simulink model "Foc"  (R2025b)
settings: Solver=FixedStepDiscrete  StartTime=0.0  StopTime=10.0  FixedStep=0.001  RelTol=1e-3
values from neighbouring files (symbols this model uses):
  cal_bActHwMode = NoneSAR.Parameter    [Foc_2024b_LoadCalParameter.m]    (also in Foc_LoadCalParameter.m)
  cal_f32AdcMaxCountsHw = NoneSAR.Parameter    [Foc_LoadCalParameter.m]
  cal_f32AdcRefVoltHw = NoneSAR.Parameter    [Foc_LoadCalParameter.m]
  cal_f32AdcVoltMidHw = NoneSAR.Parameter    [Foc_LoadCalParameter.m]
  cal_f32FullScaleCur = NoneSAR.Parameter    [Foc_LoadCalParameter.m]
  cal_f32GainAmpHw = NoneSAR.Parameter    [Foc_LoadCalParameter.m]
  cal_f32OhmRShuntHw = NoneSAR.Parameter    [Foc_LoadCalParameter.m]
  cal_s16HwtDutyU = NoneSAR.Parameter    [Foc_LoadCalParameter.m]
  cal_s16HwtDutyV = NoneSAR.Parameter    [Foc_LoadCalParameter.m]
  cal_s16HwtDutyW = NoneSAR.Parameter    [Foc_LoadCalParameter.m]
  cal_s16IdKi = NoneSAR.Parameter    [Foc_LoadCalParameter.m]
  cal_s16IdKp = NoneSAR.Parameter    [Foc_LoadCalParameter.m]
  cal_s16IdMaxOut = NoneSAR.Parameter    [Foc_LoadCalParameter.m]
  cal_s16IdMinOut = NoneSAR.Parameter    [Foc_LoadCalParameter.m]
  cal_s16Inductivity = NoneSAR.Parameter    [Foc_2024b_LoadCalParameter.m]    (also in Foc_LoadCalParameter.m)
  cal_s16IqKi = NoneSAR.Parameter    [Foc_LoadCalParameter.m]
  cal_s16IqKp = NoneSAR.Parameter    [Foc_LoadCalParameter.m]
  cal_s16IqMaxOut = NoneSAR.Parameter    [Foc_LoadCalParameter.m]
  cal_s16IqMinOut = NoneSAR.Parameter    [Foc_LoadCalParameter.m]
  cal_s16LpfPllEst = NoneSAR.Parameter    [Foc_2024b_LoadCalParameter.m]    (also in Foc_LoadCalParameter.m)
  cal_s16LpfPllEstOpenLoop = NoneSAR.Parameter    [Foc_2024b_LoadCalParameter.m]    (also in Foc_LoadCalParameter.m)
  cal_s16MinSampleTime = NoneSAR.Parameter    [Foc_2024b_LoadCalParameter.m]    (also in Foc_LoadCalParameter.m)
  cal_s16OmegaGainEst = NoneSAR.Parameter    [Foc_2024b_LoadCalParameter.m]    (also in Foc_LoadCalParameter.m)
  cal_s16RPha = NoneSAR.Parameter    [Foc_2024b_LoadCalParameter.m]    (also in Foc_LoadCalParameter.m)
  cal_s16ThresholdPhaCurImplaisible = NoneSAR.Parameter    [Foc_2024b_LoadCalParameter.m]    (also in Foc_LoadCalParameter.m)
  cal_s8IdFacKi = NoneSAR.Parameter    [Foc_LoadCalParameter.m]
  cal_s8IdFacKp = NoneSAR.Parameter    [Foc_LoadCalParameter.m]
  cal_s8IqFacKi = NoneSAR.Parameter    [Foc_LoadCalParameter.m]
  cal_s8IqFacKp = NoneSAR.Parameter    [Foc_LoadCalParameter.m]
  cal_u16AdcTriggerOffset = NoneSAR.Parameter    [Foc_LoadCalParameter.m]
  cal_u8HwtSector = NoneSAR.Parameter    [Foc_LoadCalParameter.m]
  cal_u8TiDebPhaCur = NoneSAR.Parameter    [Foc_2024b_LoadCalParameter.m]    (also in Foc_LoadCalParameter.m)
undefined symbols (not defined in the file or in its folder): CCU6_T12PERIOD, CCU_PWM_PERIOD_TICKS_HALF, DCLINK_VOLTAGE_FACTOR, DesiredPwm_U, DesiredPwm_V, DesiredPwm_W, e_motorstate_t, e_running_dir_t, FOC_SVM_MAX, FOC_VD_VQ_MAX, FOC_VD_VQ_MAX_100, FOC_VD_VQ_MAX_95, FOC_VD_VQ_MAX_97, FOCLLD_CCU_PWM_PERIOD_TICKS_HALF, FOCLLD_SKIP_DEAD_TIME_THRESHOLD, MAX_DUTY, MIN_SAMPLE_TIME_DEFAULT, MODULATION_FLATBOTTOM, ONEBY_CURRENT_AMPLIFICATION, PhaseCurrentU, PhaseCurrentV, PhaseCurrentW, PwmShift_DutyLong, PwmShift_DutyMed, PwmShift_DutyShort, PwmShiftPtr_RiseLong, PwmShiftPtr_RiseMed, PwmShiftPtr_RiseShort, s16_EST_THETA_GAIN, s16_ONEBYSQR3, s16_SQR3OVER2, st_c_pi_Q_s16_outMax, st_c_pi_Q_s16_outMin, U8_INDUCTIVITY_FAC, VQ_MAX_TABLE_SIZE, VqMaxTable_100, VqMaxTable_95, VqMaxTable_97
libraries: simulink x16, hdlsllib x2
(part 2 of 6)

== system Foc/FieldOrientedControl/CurrentControl/MOTOR_STATE_CLOSED_LOOP ==
  s16ThetaEst : Inport  OutDataTypeStr=int16
  s16Id : Inport  Port=2  OutDataTypeStr=int16
  s16Iq : Inport  Port=3  OutDataTypeStr=int16
  bEnMotorDriverLast : Inport  Port=4  OutDataTypeStr=boolean
  s16IdRef : Inport  Port=5  OutDataTypeStr=int16
  s16IqRef : Inport  Port=6  OutDataTypeStr=int16
  IqPiBus : Inport  Port=7
  IdPiBus : Inport  Port=8
  " PiCtrl_Calc" : Subsystem
  Bus Creator : BusCreator  Inputs=4
  PIControl_update : Subsystem
  foc_state : Outport
  wires:
  Bus Creator/1 -> foc_state/1
  s16Id/1 -> " PiCtrl_Calc"/1(s16Id)
  s16Iq/1 -> PIControl_update/1(s16Iq)
  PIControl_update/1(s16Vq) -> Bus Creator/3  "s16Vq"
  s16ThetaEst/1 -> Bus Creator/1  "s16_foc_parkangle"
  " PiCtrl_Calc"/1(s16Vd) -> Bus Creator/2  "s16Vd"
  bEnMotorDriverLast/1 -> Bus Creator/4  "bEnMotorDriver"
  s16IdRef/1 -> " PiCtrl_Calc"/2(s16IdRef)
  IdPiBus/1 -> " PiCtrl_Calc"/3(IdPiBus)
  s16IqRef/1 -> PIControl_update/2(s16IqRef)
  IqPiBus/1 -> PIControl_update/3(IqPiBus)

== system Foc/FieldOrientedControl/CurrentControl/MOTOR_STATE_RAMP ==
  eDirRun : Inport
  s16AngleParkLast : Inport  Port=2  OutDataTypeStr=int16
  s16Id : Inport  Port=3  OutDataTypeStr=int16
  s16Iq : Inport  Port=4  OutDataTypeStr=int16
  bEnMotorDriverLast : Inport  Port=5  OutDataTypeStr=boolean
  u32SpdRamp : Inport  Port=6  OutDataTypeStr=uint32
  s16IdRef : Inport  Port=7  OutDataTypeStr=int16
  s16IqRef : Inport  Port=8  OutDataTypeStr=int16
  IqPiBus : Inport  Port=9
  IdPiBus : Inport  Port=10
  Bus Creator : BusCreator  Inputs=4
  PiCtrl_Calc_D : Subsystem
  "PiCtrl_Calc_Q " : Subsystem
  parkangle_cal : Subsystem
  foc_state : Outport
  wires:
  eDirRun/1 -> parkangle_cal/1(eDirRun)
  u32SpdRamp/1 -> parkangle_cal/2(u32SpdRamp)
  PiCtrl_Calc_D/1(s16Vd) -> Bus Creator/2  "s16_foc_v_d"
  s16AngleParkLast/1 -> parkangle_cal/3(s16AngleParkLast)
  s16Id/1 -> PiCtrl_Calc_D/1(s16Id)
  parkangle_cal/1(s16AnglePark) -> Bus Creator/1  "s16_foc_parkangle"
  s16Iq/1 -> "PiCtrl_Calc_Q "/1(s16Iq)
  "PiCtrl_Calc_Q "/1(s16Vq) -> Bus Creator/3  "s16_foc_v_q"
  bEnMotorDriverLast/1 -> Bus Creator/4  "bEnMotorDriver"
  Bus Creator/1 -> foc_state/1
  s16IdRef/1 -> PiCtrl_Calc_D/2(s16IdRef)
  IdPiBus/1 -> PiCtrl_Calc_D/3(IdPiBus)
  s16IqRef/1 -> "PiCtrl_Calc_Q "/2(s16IqRef)
  IqPiBus/1 -> "PiCtrl_Calc_Q "/3(IqPiBus)

== system Foc/FieldOrientedControl/CurrentControl/MOTOR_STATE_RAMP_INIT ==
  s16AngleParkLast : Inport  OutDataTypeStr=int16
  s16Id : Inport  Port=2  OutDataTypeStr=int16
  s16Iq : Inport  Port=3  OutDataTypeStr=int16
  bEnMotorDriverLast : Inport  Port=4  OutDataTypeStr=boolean
  s16IdRef : Inport  Port=5  OutDataTypeStr=int16
  s16IqRef : Inport  Port=6  OutDataTypeStr=int16
  IqPiBus : Inport  Port=7
  IdPiBus : Inport  Port=8
  Compare To Constant : simulink/Logic and Bit Operations/Compare To Constant  relop===  const=false  OutDataTypeStr=boolean
  EnableDriver : Subsystem
  SetPiController : Subsystem
  Switch : Switch  Criteria=u2 ~= 0  SaturateOnIntegerOverflow=off  InputSameDT=off
  foc_state : Outport
  wires:
  s16AngleParkLast/1 -> EnableDriver/1(s16AngleParkLast)
  s16Id/1 -> SetPiController/1(s16Id)
  bEnMotorDriverLast/1 -> SetPiController/3(bEnMotorDriverLast), Compare To Constant/1
  s16Iq/1 -> SetPiController/2(s16Iq)
  EnableDriver/1(foc_state) -> Switch/1
  Compare To Constant/1 -> Switch/2
  SetPiController/1(foc_state) -> Switch/3
  Switch/1 -> foc_state/1
  s16IdRef/1 -> SetPiController/4(s16IdRef)
  IdPiBus/1 -> SetPiController/7(IdPiBus)
  s16IqRef/1 -> SetPiController/5(s16IqRef)
  IqPiBus/1 -> SetPiController/6(IqPiBus)

== system Foc/FieldOrientedControl/CurrentControl/default ==
  bEnMotorDriverLast : Inport  OutDataTypeStr=boolean
  Bus Creator : BusCreator  Inputs=4
  Constant : Constant  Value=0  OutDataTypeStr=fixdt(1,16,15)
  Constant1 : Constant  Value=0  OutDataTypeStr=fixdt(1,16,15)
  Constant2 : Constant  Value=0  OutDataTypeStr=fixdt(1,16,15)
  foc_state : Outport
  wires:
  Constant/1 -> Bus Creator/1  "s16AnglePark"
  Constant1/1 -> Bus Creator/2  "s16Vd"
  Constant2/1 -> Bus Creator/3  "s16Vq"
  bEnMotorDriverLast/1 -> Bus Creator/4  "bEnMotorDriver"
  Bus Creator/1 -> foc_state/1

== system Foc/FieldOrientedControl/CurrentOffsets/OffsetDefault ==
  Action Port : ActionPort  ActionPortLabel=else
  Constant1 : Constant  Value=0  OutDataTypeStr=int32
  Constant2 : Constant  Value=0  OutDataTypeStr=int16
  Constant3 : Constant  Value=0  OutDataTypeStr=int16
  Constant4 : Constant  Value=0  OutDataTypeStr=int32
  s16PhaCurU : Outport  OutDataTypeStr=int16
  s16PhaCurV : Outport  Port=2  OutDataTypeStr=int16
  s32CurOffsetU : Outport  Port=3  OutDataTypeStr=int32
  s32CurOffsetV : Outport  Port=4  OutDataTypeStr=int32
  wires:
  Constant3/1 -> s16PhaCurV/1
  Constant4/1 -> s32CurOffsetV/1
  Constant1/1 -> s32CurOffsetU/1
  Constant2/1 -> s16PhaCurU/1

== system Foc/FieldOrientedControl/CurrentOffsets/OffsetDetection ==
  s16PhaCurRawU : Inport  OutDataTypeStr=int16
  s16PhaCurRawV : Inport  Port=2  OutDataTypeStr=int16
  s32CurOffsetULast : Inport  Port=3  OutDataTypeStr=int32
  s32CurOffsetVLast : Inport  Port=4  OutDataTypeStr=int32
  Action Port : ActionPort  ActionPortLabel=if(u1)
  Add : Sum  Inputs=+-  OutDataTypeStr=fixdt(1,16,15)
  Add1 : Sum  Inputs=+-  OutDataTypeStr=fixdt(1,16,15)
  Add2 : Sum  OutDataTypeStr=int32
  Add3 : Sum  OutDataTypeStr=int32
  Bit Shift : hdlsllib/Logic and Bit Operations/Bit Shift  mode=Shift Right Logical  N=16
  Bit Shift1 : hdlsllib/Logic and Bit Operations/Bit Shift  mode=Shift Right Logical  N=16
  Data Type Conversion : DataTypeConversion  OutDataTypeStr=int16  SaturateOnIntegerOverflow=off  RndMeth=Floor
  Data Type Conversion1 : DataTypeConversion  OutDataTypeStr=int16  SaturateOnIntegerOverflow=off  RndMeth=Floor
  s16PhaCurU : Outport  OutDataTypeStr=int16
  s16PhaCurV : Outport  Port=2  OutDataTypeStr=int16
  s32CurOffsetU : Outport  Port=3  OutDataTypeStr=int32
  s32CurOffsetV : Outport  Port=4  OutDataTypeStr=int32
  wires:
  s32CurOffsetVLast/1 -> Add3/2, Bit Shift1/1
  s16PhaCurRawV/1 -> Add1/1
  s32CurOffsetULast/1 -> Add2/2, Bit Shift/1
  s16PhaCurRawU/1 -> Add/1
  Bit Shift/1 -> Data Type Conversion1/1
  Data Type Conversion/1 -> Add1/2
  Data Type Conversion1/1 -> Add/2
  Bit Shift1/1 -> Data Type Conversion/1
  Add3/1 -> s32CurOffsetV/1
  Add2/1 -> s32CurOffsetU/1
  Add1/1 -> Add3/1, s16PhaCurV/1
  Add/1 -> s16PhaCurU/1, Add2/1

== system Foc/FieldOrientedControl/GetCurrents/AdcVolToCur ==
  u16SsCur1 : Inport  OutDataTypeStr=uint16
  u16SsCur2 : Inport  Port=2  OutDataTypeStr=uint16
  Add : Sum  Inputs=+-
  Add1 : Sum
  Add2 : Sum  Inputs=+-
  Add3 : Sum
  Constant : Constant  Value=cal_f32AdcMaxCountsHw  OutDataTypeStr=single
  Constant1 : Constant  Value=cal_f32AdcRefVoltHw  OutDataTypeStr=single
  Constant10 : Constant  Value=cal_f32AdcRefVoltHw  OutDataTypeStr=single
  Constant11 : Constant  Value=cal_f32OhmRShuntHw  OutDataTypeStr=single
  Constant12 : Constant  Value=cal_f32GainAmpHw  OutDataTypeStr=single
  Constant13 : Constant  Value=cal_f32AdcVoltMidHw  OutDataTypeStr=single
  Constant14 : Constant  Value=0.5  OutDataTypeStr=single
  Constant15 : Constant  Value=-0.5  OutDataTypeStr=single
  Constant16 : Constant  Value=32767  OutDataTypeStr=single
  Constant17 : Constant  Value=cal_f32FullScaleCur  OutDataTypeStr=single
  Constant2 : Constant  Value=cal_f32OhmRShuntHw  OutDataTypeStr=single
  Constant3 : Constant  Value=cal_f32GainAmpHw  OutDataTypeStr=single
  Constant4 : Constant  Value=cal_f32AdcVoltMidHw  OutDataTypeStr=single
  Constant5 : Constant  Value=0.5  OutDataTypeStr=single
  Constant6 : Constant  Value=-0.5  OutDataTypeStr=single
  Constant7 : Constant  Value=32767  OutDataTypeStr=single
  Constant8 : Constant  Value=cal_f32FullScaleCur  OutDataTypeStr=single
  Constant9 : Constant  Value=cal_f32AdcMaxCountsHw  OutDataTypeStr=single
  Data Type Conversion : DataTypeConversion  OutDataTypeStr=single  SaturateOnIntegerOverflow=off  RndMeth=Floor
  Data Type Conversion1 : DataTypeConversion  OutDataTypeStr=single  SaturateOnIntegerOverflow=off  RndMeth=Floor
  Data Type Conversion : DataTypeConversion  OutDataTypeStr=int32  SaturateOnIntegerOverflow=off  RndMeth=Floor
  Data Type Conversion1 : DataTypeConversion  OutDataTypeStr=int32  SaturateOnIntegerOverflow=off  RndMeth=Floor
  Divide{,3..4,6,9..10} (6 alike) : Product  Inputs=*/
  Divide{1..2,5,7..8,11} (6 alike) : Product  Inputs=**
  Saturation : Saturate  UpperLimit=32767  LowerLimit=-32768  OutDataTypeStr=int16
  Saturation1 : Saturate  UpperLimit=32767  LowerLimit=-32768  OutDataTypeStr=int16
  Switch : Switch  Criteria=u2 > Threshold  SaturateOnIntegerOverflow=off  InputSameDT=off
  Switch1 : Switch  Criteria=u2 > Threshold  SaturateOnIntegerOverflow=off  InputSameDT=off
  s16SsCur1 : Outport  OutDataTypeStr=int16
  s16SsCur2 : Outport  Port=2  OutDataTypeStr=int16
  wires:
  u16SsCur1/1 -> Data Type Conversion/1
  Add1/1 -> Data Type Conversion/1
  Add3/1 -> Data Type Conversion1/1
  u16SsCur2/1 -> Data Type Conversion1/1
  Data Type Conversion/1 -> Divide/1
  Divide10/1 -> Divide11/1
  Divide/1 -> Divide1/1
  Constant9/1 -> Divide6/2
  Constant8/1 -> Divide4/2
  Data Type Conversion1/1 -> Divide6/1
  Constant6/1 -> Switch/3
  Constant14/1 -> Switch1/1
  Constant2/1 -> Divide2/1
  Constant10/1 -> Divide7/2
  Constant16/1 -> Divide11/2
  Constant4/1 -> Add/2
  Constant12/1 -> Divide8/2
  Constant/1 -> Divide/2
  Divide4/1 -> Divide5/1
  Divide2/1 -> Divide3/2
  Divide8/1 -> Divide9/2
  Divide6/1 -> Divide7/1
  Constant5/1 -> Switch/1
  Constant17/1 -> Divide10/2
  Constant13/1 -> Add2/2
  Constant1/1 -> Divide1/2
  Divide5/1 -> Add1/2
  Divide3/1 -> Divide4/1, Switch/2
  Divide9/1 -> Switch1/2, Divide10/1
  Divide7/1 -> Add2/1
  Constant7/1 -> Divide5/2
  Constant15/1 -> Switch1/3
  Constant3/1 -> Divide2/2
  Constant11/1 -> Divide8/1
  Data Type Conversion1/1 -> Saturation1/1
  Divide11/1 -> Add3/2
  Divide1/1 -> Add/1
  Add/1 -> Divide3/1
  Add2/1 -> Divide9/1
  Switch1/1 -> Add3/1
  Saturation/1 -> s16SsCur1/1
  Switch/1 -> Add1/1
  Data Type Conversion/1 -> Saturation/1
  Saturation1/1 -> s16SsCur2/1

== system Foc/FieldOrientedControl/GetCurrents/DEFAULT ==
  Action Port : ActionPort
  Constant : Constant  Value=0  OutDataTypeStr=int16
  Constant1 : Constant  Value=0  OutDataTypeStr=int16
  Constant2 : Constant  Value=0  OutDataTypeStr=int16
  s16PhaCurU : Outport  OutDataTypeStr=int16
  s16PhaCurV : Outport  Port=2  OutDataTypeStr=int16
  s16PhaCurW : Outport  Port=3  OutDataTypeStr=int16
  wires:
  Constant1/1 -> s16PhaCurV/1
  Constant/1 -> s16PhaCurW/1
  Constant2/1 -> s16PhaCurU/1

== system Foc/FieldOrientedControl/GetCurrents/SECTOR_1 ==
  s16SsCur1 : Inport  OutDataTypeStr=int16
  s16SsCur2 : Inport  Port=2  OutDataTypeStr=int16
  Action Port : ActionPort
  Add : Sum  Inputs=+-  OutDataTypeStr=fixdt(1,16,15)
  Constant : Constant  Value=-1  OutDataTypeStr=int16
  Gain : Gain  Gain=-1
  Product : Product  OutDataTypeStr=fixdt(1,16,15)
  s16PhaCurU : Outport  OutDataTypeStr=int16
  s16PhaCurV : Outport  Port=2  OutDataTypeStr=int16
  s16PhaCurW : Outport  Port=3  OutDataTypeStr=int16
  wires:
  Add/1 -> s16PhaCurU/1
  Product/1 -> Add/2, s16PhaCurW/1
  Gain/1 -> Add/1
  Constant/1 -> Product/2
  s16SsCur2/1 -> Product/1
  s16SsCur1/1 -> Gain/1, s16PhaCurV/1

== system Foc/FieldOrientedControl/GetCurrents/SECTOR_2 ==
  s16SsCur1 : Inport  OutDataTypeStr=int16
  s16SsCur2 : Inport  Port=2  OutDataTypeStr=int16
  Action Port : ActionPort
  Add : Sum  Inputs=+-  OutDataTypeStr=fixdt(1,16,15)
  Constant : Constant  Value=-1  OutDataTypeStr=int16
  Gain : Gain  Gain=-1
  Product : Product  OutDataTypeStr=fixdt(1,16,15)
  s16PhaCurU : Outport  OutDataTypeStr=int16
  s16PhaCurV : Outport  Port=2  OutDataTypeStr=int16
  s16PhaCurW : Outport  Port=3  OutDataTypeStr=int16
  wires:
  Add/1 -> s16PhaCurW/1
  s16SsCur2/1 -> Product/1
  s16SsCur1/1 -> s16PhaCurU/1, Gain/1
  Product/1 -> s16PhaCurV/1, Add/2
  Gain/1 -> Add/1
  Constant/1 -> Product/2

== system Foc/FieldOrientedControl/GetCurrents/SECTOR_3 ==
  s16SsCur1 : Inport  OutDataTypeStr=int16
  s16SsCur2 : Inport  Port=2  OutDataTypeStr=int16
  Action Port : ActionPort
  Add : Sum  Inputs=+-  OutDataTypeStr=fixdt(1,16,15)
  Constant : Constant  Value=-1  OutDataTypeStr=int16
  Gain : Gain  Gain=-1
  Product : Product  OutDataTypeStr=fixdt(1,16,15)
  s16PhaCurU : Outport  OutDataTypeStr=int16
  s16PhaCurV : Outport  Port=2  OutDataTypeStr=int16
  s16PhaCurW : Outport  Port=3  OutDataTypeStr=int16
  wires:
  Product/1 -> s16PhaCurW/1, Add/2
  Gain/1 -> Add/1
  s16SsCur2/1 -> Product/1
  s16SsCur1/1 -> Gain/1, s16PhaCurU/1
  Add/1 -> s16PhaCurV/1
  Constant/1 -> Product/2

== system Foc/FieldOrientedControl/GetCurrents/SECTOR_4 ==
  s16SsCur1 : Inport  OutDataTypeStr=int16
  s16SsCur2 : Inport  Port=2  OutDataTypeStr=int16
  Action Port : ActionPort
  Add : Sum  Inputs=+-  OutDataTypeStr=fixdt(1,16,15)
  Constant : Constant  Value=-1  OutDataTypeStr=int16
  Gain : Gain  Gain=-1
  Product : Product  OutDataTypeStr=fixdt(1,16,15)
  s16PhaCurU : Outport  OutDataTypeStr=int16
  s16PhaCurV : Outport  Port=2  OutDataTypeStr=int16
  s16PhaCurW : Outport  Port=3  OutDataTypeStr=int16
  wires:
  Product/1 -> s16PhaCurU/1, Add/2
  Gain/1 -> Add/1
  s16SsCur2/1 -> Product/1
  s16SsCur1/1 -> s16PhaCurW/1, Gain/1
  Add/1 -> s16PhaCurV/1
  Constant/1 -> Product/2

== system Foc/FieldOrientedControl/GetCurrents/SECTOR_5 ==
  s16SsCur1 : Inport  OutDataTypeStr=int16
  s16SsCur2 : Inport  Port=2  OutDataTypeStr=int16
  Action Port : ActionPort
  Add : Sum  Inputs=+-  OutDataTypeStr=fixdt(1,16,15)
  Constant : Constant  Value=-1  OutDataTypeStr=int16
  Gain : Gain  Gain=-1
  Product : Product  OutDataTypeStr=fixdt(1,16,15)
  s16PhaCurU : Outport  OutDataTypeStr=int16
  s16PhaCurV : Outport  Port=2  OutDataTypeStr=int16
  s16PhaCurW : Outport  Port=3  OutDataTypeStr=int16
  wires:
  Product/1 -> Add/2, s16PhaCurU/1
  Gain/1 -> Add/1
  s16SsCur2/1 -> Product/1
  s16SsCur1/1 -> s16PhaCurV/1, Gain/1
  Add/1 -> s16PhaCurW/1
  Constant/1 -> Product/2

== system Foc/FieldOrientedControl/GetCurrents/SECTOR_6 ==
  s16SsCur1 : Inport  OutDataTypeStr=int16
  s16SsCur2 : Inport  Port=2  OutDataTypeStr=int16
  Action Port : ActionPort
  Add : Sum  Inputs=+-  OutDataTypeStr=fixdt(1,16,15)
  Constant : Constant  Value=-1  OutDataTypeStr=int16
  Gain : Gain  Gain=-1
  Product : Product  OutDataTypeStr=fixdt(1,16,15)
  s16PhaCurU : Outport  OutDataTypeStr=int16
  s16PhaCurV : Outport  Port=2  OutDataTypeStr=int16
  s16PhaCurW : Outport  Port=3  OutDataTypeStr=int16
  wires:
  s16SsCur2/1 -> Product/1
  s16SsCur1/1 -> s16PhaCurW/1, Gain/1
  Add/1 -> s16PhaCurU/1
  Constant/1 -> Product/2
  Product/1 -> s16PhaCurV/1, Add/2
  Gain/1 -> Add/1

== system Foc/FieldOrientedControl/PhaseCurrentSpikeMonitor/b_fault_debounce  ==
  bSymptom : Inport  OutDataTypeStr=boolean
  u8TiDeb : Inport  Port=2  OutDataTypeStr=uint8
  Add : Sum
  CNST_ONE : Constant  OutDataTypeStr=uint8
  CNST_Thd : Constant  Value=200
  CNST_Thd1 : Constant  Value=200
  CNST_Zero : Constant  Value=0
  CNST_flase : Constant  Value=false  OutDataTypeStr=boolean
  CNST_true : Constant  Value=true  OutDataTypeStr=boolean
  DLY_timer : UnitDelay  SampleTime=-1  HasFrameUpgradeWarning=on
  Relational Operator : RelationalOperator  Operator=<  OutDataTypeStr=boolean  RndMeth=Simplest  InputSameDT=off
  Relational Operator1 : RelationalOperator  OutDataTypeStr=boolean  RndMeth=Simplest  InputSameDT=off
  Switch1 : Switch  Criteria=u2 ~= 0  SaturateOnIntegerOverflow=off  InputSameDT=off
  Switch2 : Switch  Criteria=u2 ~= 0  SaturateOnIntegerOverflow=off  InputSameDT=off
  Switch3 : Switch  Criteria=u2 ~= 0  SaturateOnIntegerOverflow=off  InputSameDT=off
  bFlgFlt : Outport  OutDataTypeStr=boolean
  wires:
  CNST_Thd/1 -> Relational Operator/2
  CNST_Zero/1 -> Switch2/3
  CNST_flase/1 -> Switch1/3
  bSymptom/1 -> Switch2/2
  Add/1 -> Switch2/1
  CNST_ONE/1 -> Add/2
  Relational Operator/1 -> Switch3/2
  Switch2/1 -> Relational Operator/1, Switch3/1, DLY_timer/1
  DLY_timer/1 -> Add/1
  Switch3/1 -> Relational Operator1/1
  CNST_Thd1/1 -> Switch3/3
  Switch1/1 -> bFlgFlt/1
  CNST_true/1 -> Switch1/1
  u8TiDeb/1 -> Relational Operator1/2
  Relational Operator1/1 -> Switch1/2

== system Foc/FieldOrientedControl/PllObserver/BackEMF ==
  s16VGainEst : Inport  OutDataTypeStr=int16
  s16IAlpha : Inport  Port=2  OutDataTypeStr=int16
  s16VAlphaLast : Inport  Port=3  OutDataTypeStr=int16
  s16IBeta : Inport  Port=4  OutDataTypeStr=int16
  s16VBetaLast : Inport  Port=5  OutDataTypeStr=int16
  AlphaBackEMF : Subsystem  Description=|
      | Back EMF calculation for e_alpha
      | e = v - i * R - di/dt * L
      | calculate term -di/dt * L = (i(n) - i(n-1)) * (-L) * scaling factor
      | calculate term i*R, and then calculate v - i*R - di/dt * L, v is scaled with s16_est_vigain
  BetaBackEMF : Subsystem  Description=|
      | Back EMF calculation for e_beta
      | e = v - i * R - di/dt * L
      | calculate term -di/dt * L = (i(n) - i(n-1)) * (-L) * scaling factor
      | calculate term i*R, and then calculate v - i*R - di/dt * L, v is scaled with s16_est_vigain
  s16VGainEst1 : InportShadow  OutDataTypeStr=int16
  s16LAlphaEst : Outport  OutDataTypeStr=int16
  s16LBetaEst : Outport  Port=2  OutDataTypeStr=int16
  s16EAlphaEst : Outport  Port=3  OutDataTypeStr=int16
  s16EBetaEst : Outport  Port=4  OutDataTypeStr=int16
  wires:
  s16VBetaLast/1 -> BetaBackEMF/2(s16VBetaLast)
  s16IBeta/1 -> BetaBackEMF/1(s16IBeta)
  s16VGainEst/1 -> AlphaBackEMF/3(s16VGainEst)
  s16VAlphaLast/1 -> AlphaBackEMF/2(s16VAlphaLast)
  s16IAlpha/1 -> AlphaBackEMF/1(s16IAlpha)
  s16VGainEst1/1 -> BetaBackEMF/3(s16VGainEst)
  AlphaBackEMF/1(s16LAlphaEst) -> s16LAlphaEst/1
  AlphaBackEMF/2(s16EAlphaEst) -> s16EAlphaEst/1
  BetaBackEMF/1(s16LBetaEst) -> s16LBetaEst/1
  BetaBackEMF/2(s16EBetaEst) -> s16EBetaEst/1

== system Foc/FieldOrientedControl/PllObserver/LowPassFilter ==
  s16EdEst : Inport  OutDataTypeStr=int16
  s16EqEst : Inport  Port=2  OutDataTypeStr=int16
  eStMotor : Inport  Port=3
  Add{8,10,12,14} (4 alike) : Sum  Inputs=+-
  Add{9,11,13,15} (4 alike) : Sum  OutDataTypeStr=fixdt(1,16,15)
  Constant14 : Constant  Value=cal_s16LpfPllEst  OutDataTypeStr=int16
  Constant16 : Constant  Value=cal_s16LpfPllEst  OutDataTypeStr=int16
  Constant17 : Constant  Value=cal_s16LpfPllEstOpenLoop  OutDataTypeStr=int16
  Constant18 : Constant  Value=cal_s16LpfPllEstOpenLoop  OutDataTypeStr=int16
  Enumerated Constant1 : simulink/Sources/Enumerated Constant  OutDataTypeStr=Enum: e_motorstate_t  Value=e_motorstate_t.MOTOR_STATE_CLOSED_LOOP  SampleTime=inf
  Enumerated Constant2 : simulink/Sources/Enumerated Constant  OutDataTypeStr=Enum: e_motorstate_t  Value=e_motorstate_t.MOTOR_STATE_CLOSED_LOOP  SampleTime=inf
  Product{15..18} (4 alike) : Product
  Relational Operator1 : RelationalOperator  Operator===  OutDataTypeStr=boolean  RndMeth=Simplest  InputSameDT=off
  Relational Operator2 : RelationalOperator  Operator===  OutDataTypeStr=boolean  RndMeth=Simplest  InputSameDT=off
  Switch2 : Switch  Criteria=u2 ~= 0  SaturateOnIntegerOverflow=off  InputSameDT=off
  Switch3 : Switch  Criteria=u2 ~= 0  SaturateOnIntegerOverflow=off  InputSameDT=off
  Unit Delay2 : UnitDelay  SampleTime=-1  HasFrameUpgradeWarning=on
  Unit Delay3 : UnitDelay  SampleTime=-1  HasFrameUpgradeWarning=on
  eStMotor1 : InportShadow  Port=3
  s16EdEst1 : InportShadow  OutDataTypeStr=int16
  s16EqEst1 : InportShadow  Port=2  OutDataTypeStr=int16
  s16EqFilterEst : Outport  OutDataTypeStr=int16
  s16EdFilterEst : Outport  Port=2  OutDataTypeStr=int16
  wires:
  Constant14/1 -> Product15/2
  [s16EdFilterEst] -> Add13/2, Add12/2
  Add13/1 -> Switch3/3
  Add9/1 -> Switch2/1
  eStMotor/1 -> Relational Operator2/1
  [s16EdFilterEst] -> Add11/2, Add10/2
  Enumerated Constant2/1 -> Relational Operator2/2
  Add12/1 -> Product17/1
  Add8/1 -> Product15/1
  s16EdEst/1 -> Add10/1
  Constant16/1 -> Product16/2
  Add10/1 -> Product16/1
  Add14/1 -> Product18/1
  [s16EdFilterEst] -> Add15/2, Add14/2
  s16EqEst/1 -> Add8/1
  [s16EqFilterEst] -> Add9/2, Add8/2
  s16EqEst1/1 -> Add14/1
  Product17/1 -> Add13/1
  s16EdEst1/1 -> Add12/1
  Add11/1 -> Switch3/1
  Add15/1 -> Switch2/3
  Constant18/1 -> Product18/2
  Constant17/1 -> Product17/2
  Product15/1 -> Add9/1
  eStMotor1/1 -> Relational Operator1/1
  Enumerated Constant1/1 -> Relational Operator1/2
  Product18/1 -> Add15/1
  Unit Delay3/1 -> [s16EdFilterEst]
  Product16/1 -> Add11/1
  Relational Operator1/1 -> Switch2/2
  Relational Operator2/1 -> Switch3/2
  Switch2/1 -> Unit Delay2/1, s16EqFilterEst/1
  Switch3/1 -> s16EdFilterEst/1, Unit Delay3/1
  Unit Delay2/1 -> [s16EqFilterEst]

== system Foc/FieldOrientedControl/PllObserver/ParkTransformationBEMF ==
  s16EAlphaEst : Inport  OutDataTypeStr=int16
  s16EBetaEst : Inport  Port=2  OutDataTypeStr=int16
  s16ThetaSinPll : Inport  Port=3  OutDataTypeStr=int16
  s16ThetaCosPll : Inport  Port=4  OutDataTypeStr=int16
  Add6 : Sum  OutDataTypeStr=fixdt(1,16,15)
  Add7 : Sum  Inputs=+-
  Product{11..14} (4 alike) : Product  OutDataTypeStr=int16
  s16EAlphaEst1 : InportShadow  OutDataTypeStr=int16
  s16EBetaEst1 : InportShadow  Port=2  OutDataTypeStr=int16
  s16ThetaCosPll1 : InportShadow  Port=4  OutDataTypeStr=int16
  s16ThetaSinPll1 : InportShadow  Port=3  OutDataTypeStr=int16
  s16EdEst : Outport  OutDataTypeStr=int16
  s16EqEst : Outport  Port=2  OutDataTypeStr=int16
  wires:
  s16ThetaCosPll/1 -> Product12/1
  s16EBetaEst/1 -> Product11/1
  s16EAlphaEst/1 -> Product12/2
  s16ThetaSinPll/1 -> Product11/2
  s16ThetaSinPll1/1 -> Product14/1
  s16EBetaEst1/1 -> Product13/1
  s16EAlphaEst1/1 -> Product14/2
  s16ThetaCosPll1/1 -> Product13/2
  Product11/1 -> Add6/1
  Product12/1 -> Add6/2
  Product13/1 -> Add7/1
  Product14/1 -> Add7/2
  Add6/1 -> s16EdEst/1
  Add7/1 -> s16EqEst/1

== system Foc/FieldOrientedControl/PllObserver/SinCosCalculation ==
  eStMotor : Inport
  s16ThetaEst : Inport  Port=2  OutDataTypeStr=int16
  s16ThetaSin : Inport  Port=3  OutDataTypeStr=int16
  s16ThetaCos : Inport  Port=4  OutDataTypeStr=int16
  1-D Lookup Table : Lookup_n-D  NumberOfTableDimensions=1  BreakpointsForDimension1=[-5:5]  IndexSearchMethod=Linear search  Table=tanh([-5:5])  ExtrapMethod=Clip  InternalRulePriority=Speed  RndMeth=Simplest
  1-D Lookup Table1 : Lookup_n-D  NumberOfTableDimensions=1  BreakpointsForDimension1=[-5:5]  Table=tanh([-5:5])  ExtrapMethod=Clip  InternalRulePriority=Speed  RndMeth=Simplest
  Demux : Demux  Outputs=2
  Enumerated Constant3 : simulink/Sources/Enumerated Constant  OutDataTypeStr=Enum: e_motorstate_t  Value=e_motorstate_t.MOTOR_STATE_RAMP  SampleTime=inf
  Mux1 : Mux  Inputs=2
  Mux2 : Mux  Inputs=2
  Relational Operator : RelationalOperator  Operator===  OutDataTypeStr=boolean  RndMeth=Simplest  InputSameDT=off
  Switch : Switch  Criteria=u2 ~= 0  SaturateOnIntegerOverflow=off  InputSameDT=off
  s16ThetaSinPll : Outport  OutDataTypeStr=int16
  s16ThetaCosPll : Outport  Port=2  OutDataTypeStr=int16
  wires:
  s16ThetaCos/1 -> Mux2/2
  Enumerated Constant3/1 -> Relational Operator/2
  1-D Lookup Table1/1 -> Mux1/2
  s16ThetaEst/1 -> 1-D Lookup Table/1, 1-D Lookup Table1/1
  1-D Lookup Table/1 -> Mux1/1
  Mux1/1 -> Switch/1
  s16ThetaSin/1 -> Mux2/1
  eStMotor/1 -> Relational Operator/1
  Relational Operator/1 -> Switch/2
  Mux2/1 -> Switch/3
  Switch/1 -> Demux/1
  Demux/1 -> s16ThetaSinPll/1
  Demux/2 -> s16ThetaCosPll/1

== system Foc/FieldOrientedControl/PllObserver/SupplyVoltageAdaptive ==
  u16DcLinkVoltage : Inport  OutDataTypeStr=uint16
  Add22 : Sum  OutDataTypeStr=uint16
  Constant : Constant  Value=ONEBY_CURRENT_AMPLIFICATION  OutDataTypeStr=int16
  Constant1 : Constant  Value=DCLINK_VOLTAGE_FACTOR  OutDataTypeStr=fixdt(1,16,15)
  Constant2 : Constant  Value=2  OutDataTypeStr=uint8
  Constant3 : Constant  Value=5.0  OutDataTypeStr=single
  Constant32 : Constant  Value=0.5  OutDataTypeStr=single
  Constant4 : Constant  Value=4095.0  OutDataTypeStr=single
  Constant5 : Constant  Value=10.0  OutDataTypeStr=single
  Constant6 : Constant  Value=43.0  OutDataTypeStr=single
  Constant7 : Constant  Value=10.0  OutDataTypeStr=single
  Constant8 : Constant  Value=10.0  OutDataTypeStr=single
  Data Type Conversion : DataTypeConversion  OutDataTypeStr=single  SaturateOnIntegerOverflow=off  RndMeth=Floor
  Data Type Conversion1 : DataTypeConversion  OutDataTypeStr=int32  SaturateOnIntegerOverflow=off  RndMeth=Floor
  Data Type Conversion2 : DataTypeConversion  OutDataTypeStr=int16  SaturateOnIntegerOverflow=off  RndMeth=Floor
  Data Type Conversion3 : DataTypeConversion  OutDataTypeStr=uint8  SaturateOnIntegerOverflow=off  RndMeth=Floor
  Data Type Conversion4 : DataTypeConversion  OutDataTypeStr=uint8  SaturateOnIntegerOverflow=off  RndMeth=Floor
  Data Type Conversion5 : DataTypeConversion  OutDataTypeStr=int16  SaturateOnIntegerOverflow=off  RndMeth=Floor
  Divide : Product  Inputs=*/
  Divide1 : Product  Inputs=*/  OutDataTypeStr=fixdt(1,16,15)
  Divide2 : Product  Inputs=*/
  Divide3 : Product  Inputs=*/
  Product{,1..4} (5 alike) : Product  OutDataTypeStr=int16
  s16VGainEst : Outport  OutDataTypeStr=int16
  u8VSplyCan : Outport  Port=2  OutDataTypeStr=uint8
  u16VSply : Outport  Port=3  OutDataTypeStr=uint16
  wires:
  Add22/1 -> Data Type Conversion5/1
  u16DcLinkVoltage/1 -> Data Type Conversion/1, Data Type Conversion1/1
  Constant3/1 -> Product1/1
  Constant1/1 -> Add22/1
  Product2/1 -> Data Type Conversion3/1
  Constant/1 -> Product/2
  Product/1 -> Divide/1
  Data Type Conversion1/1 -> Product/1
  Product4/1 -> Data Type Conversion4/1
  Divide/1 -> Divide1/1
  Constant32/1 -> Add22/2
  Data Type Conversion/1 -> Product1/2
  Product1/1 -> Divide2/1
  Constant4/1 -> Divide2/2
  Product3/1 -> Divide3/1
  Constant2/1 -> Divide1/2
  Data Type Conversion5/1 -> Divide/2
  Divide1/1 -> Data Type Conversion2/1
  Constant5/1 -> Product2/1
  Constant7/1 -> Divide3/2
  Divide2/1 -> Product3/1, Product2/2
  Constant6/1 -> Product3/2
  Data Type Conversion3/1 -> u8VSplyCan/1
  Constant8/1 -> Product4/1
  Divide3/1 -> Product4/2
  Data Type Conversion2/1 -> s16VGainEst/1
  Data Type Conversion4/1 -> u16VSply/1

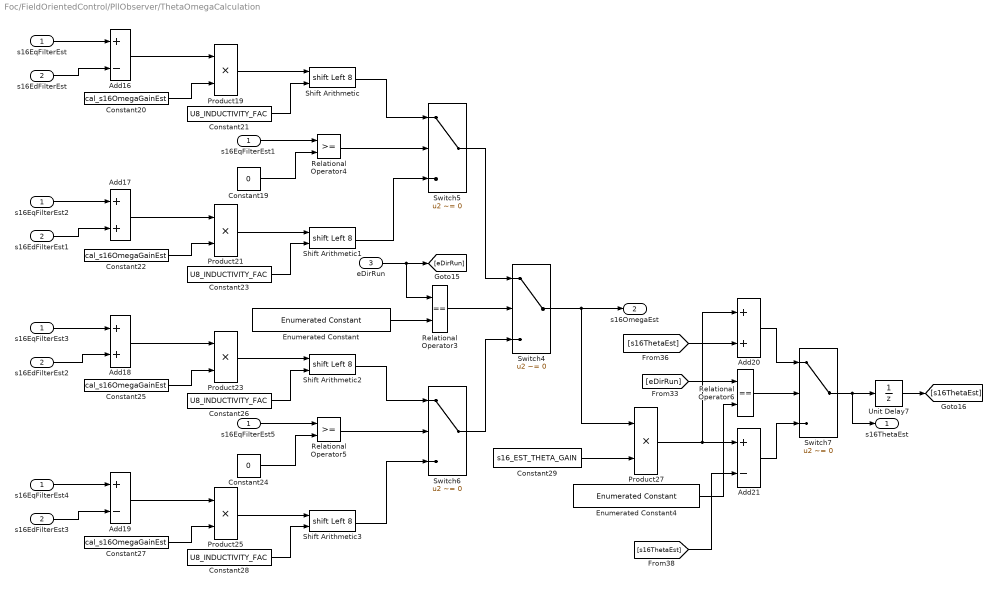
== system Foc/FieldOrientedControl/PllObserver/ThetaOmegaCalculation ==
  s16EqFilterEst : Inport  OutDataTypeStr=int16
  s16EdFilterEst : Inport  Port=2  OutDataTypeStr=int16
  eDirRun : Inport  Port=3
  Add16 : Sum  Inputs=+-
  Add17 : Sum
  Add18 : Sum
  Add19 : Sum  Inputs=+-
  Add20 : Sum  OutDataTypeStr=fixdt(1,16,15)
  Add21 : Sum  Inputs=+-  OutDataTypeStr=fixdt(1,16,15)
  Constant19 : Constant  Value=0
  Constant{20,22,25,27} (4 alike) : Constant  Value=cal_s16OmegaGainEst  OutDataTypeStr=int16
  Constant{21,23,26,28} (4 alike) : Constant  Value=U8_INDUCTIVITY_FAC  OutDataTypeStr=int16
  Constant24 : Constant  Value=0
  Constant29 : Constant  Value=s16_EST_THETA_GAIN
  Enumerated Constant : simulink/Sources/Enumerated Constant  OutDataTypeStr=Enum: e_running_dir_t  Value=e_running_dir_t.CLOCKWISE  SampleTime=inf
  Enumerated Constant4 : simulink/Sources/Enumerated Constant  OutDataTypeStr=Enum: e_running_dir_t  Value=e_running_dir_t.CLOCKWISE  SampleTime=inf
  Product{19,21,23,25} (4 alike) : Product  OutDataTypeStr=int16
  Product27 : Product  OutDataTypeStr=fixdt(1,16,15)
  Relational Operator3 : RelationalOperator  Operator===  OutDataTypeStr=boolean  RndMeth=Simplest  InputSameDT=off
  Relational Operator4 : RelationalOperator  OutDataTypeStr=boolean  RndMeth=Simplest  InputSameDT=off
  Relational Operator5 : RelationalOperator  OutDataTypeStr=boolean  RndMeth=Simplest  InputSameDT=off
  Relational Operator6 : RelationalOperator  Operator===  OutDataTypeStr=boolean  RndMeth=Simplest  InputSameDT=off
  Shift Arithmetic{,1..3} (4 alike) : ArithShift  BitShiftNumberSource=Input port  BitShiftNumber=8  BitShiftDirection=Left
      settings: InputPortMap=u0,p1
  Switch{4..7} (4 alike) : Switch  Criteria=u2 ~= 0  SaturateOnIntegerOverflow=off  InputSameDT=off
  Unit Delay7 : UnitDelay  SampleTime=-1  HasFrameUpgradeWarning=on
  s16EdFilterEst1 : InportShadow  Port=2  OutDataTypeStr=int16
  s16EdFilterEst2 : InportShadow  Port=2  OutDataTypeStr=int16
  s16EdFilterEst3 : InportShadow  Port=2  OutDataTypeStr=int16
  s16EqFilterEst{1..5} (5 alike) : InportShadow  OutDataTypeStr=int16
  s16ThetaEst : Outport  OutDataTypeStr=int16
  s16OmegaEst : Outport  Port=2  OutDataTypeStr=int16
  wires:
  s16EqFilterEst/1 -> Add16/1
  s16EdFilterEst2/1 -> Add18/2
  Add16/1 -> Product19/1
  s16EqFilterEst3/1 -> Add18/1
  s16EdFilterEst3/1 -> Add19/2
  s16EqFilterEst4/1 -> Add19/1
  s16EdFilterEst1/1 -> Add17/2
  s16EqFilterEst2/1 -> Add17/1
  s16EdFilterEst/1 -> Add16/2
  Relational Operator5/1 -> Switch6/2
  Constant20/1 -> Product19/2
  Constant26/1 -> Shift Arithmetic2/2
  Product23/1 -> Shift Arithmetic2/1
  Add17/1 -> Product21/1
  Relational Operator6/1 -> Switch7/2
  Product19/1 -> Shift Arithmetic/1
  Constant22/1 -> Product21/2
  Constant28/1 -> Shift Arithmetic3/2
  Product25/1 -> Shift Arithmetic3/1
  Add18/1 -> Product23/1
  Constant25/1 -> Product23/2
  Product27/1 -> Add20/1, Add21/1
  Enumerated Constant/1 -> Relational Operator3/2
  Add19/1 -> Product25/1
  Constant27/1 -> Product25/2
  Constant21/1 -> Shift Arithmetic/2
  eDirRun/1 -> [eDirRun], Relational Operator3/1
  s16EqFilterEst1/1 -> Relational Operator4/1
  Switch5/1 -> Switch4/1
  Constant19/1 -> Relational Operator4/2
  Switch7/1 -> Unit Delay7/1, s16ThetaEst/1
  Constant24/1 -> Relational Operator5/2
  Product21/1 -> Shift Arithmetic1/1
  Constant23/1 -> Shift Arithmetic1/2
  s16EqFilterEst5/1 -> Relational Operator5/1
  Shift Arithmetic/1 -> Switch5/1
  Add21/1 -> Switch7/3
  [s16ThetaEst] -> Add21/2
  Relational Operator4/1 -> Switch5/2
  Shift Arithmetic1/1 -> Switch5/3
  Shift Arithmetic2/1 -> Switch6/1
  Shift Arithmetic3/1 -> Switch6/3
  Add20/1 -> Switch7/1
  [eDirRun] -> Relational Operator6/1
  Relational Operator3/1 -> Switch4/2
  Switch6/1 -> Switch4/3
  Switch4/1 -> s16OmegaEst/1, Product27/1
  Constant29/1 -> Product27/2
  [s16ThetaEst] -> Add20/2
  Enumerated Constant4/1 -> Relational Operator6/2
  Unit Delay7/1 -> [s16ThetaEst]

== system Foc/FieldOrientedControl/SendCurrentToCan/Subsystem ==
  In : Inport  OutDataTypeStr=int16
  Constant : Constant  Value=32768  OutDataTypeStr=single
  Constant8 : Constant  Value=cal_f32FullScaleCur  OutDataTypeStr=single
  Divide : Product  Inputs=*/
  Divide1 : Product  Inputs=**
  Out : Outport  OutDataTypeStr=single
  wires:
  Divide1/1 -> Out/1
  Constant8/1 -> Divide1/2
  Divide/1 -> Divide1/1
  In/1 -> Divide/1
  Constant/1 -> Divide/2

== system Foc/FieldOrientedControl/SendCurrentToCan/Subsystem1 ==
  In : Inport  OutDataTypeStr=int16
  Constant : Constant  Value=32768  OutDataTypeStr=single
  Constant8 : Constant  Value=cal_f32FullScaleCur  OutDataTypeStr=single
  Divide : Product  Inputs=*/
  Divide1 : Product  Inputs=**
  Out : Outport  OutDataTypeStr=single
  wires:
  Divide1/1 -> Out/1
  Constant8/1 -> Divide1/2
  Divide/1 -> Divide1/1
  In/1 -> Divide/1
  Constant/1 -> Divide/2

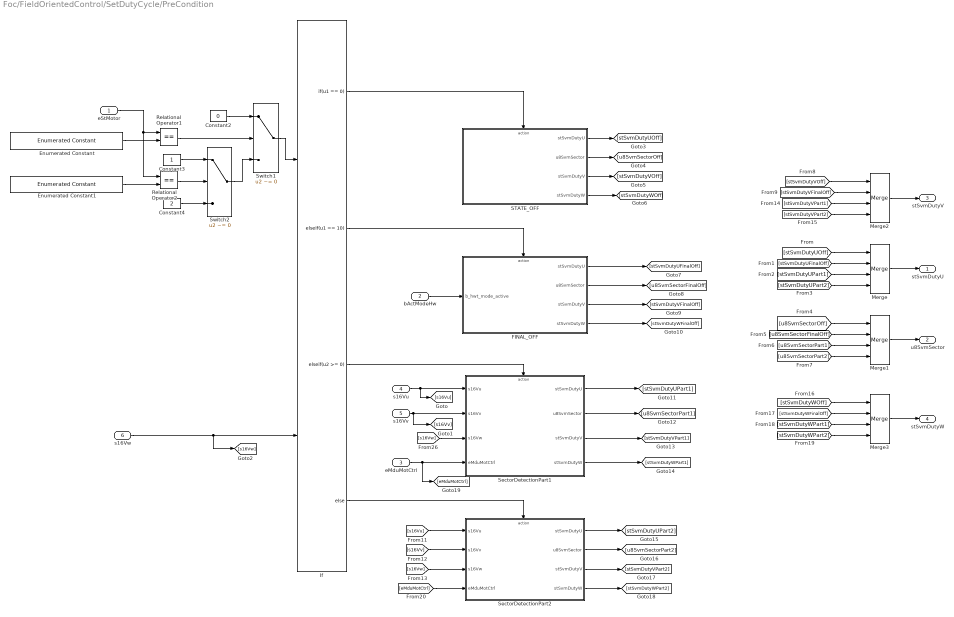
== system Foc/FieldOrientedControl/SetDutyCycle/PreCondition ==
  eStMotor : Inport
  bActModeHw : Inport  Port=2  OutDataTypeStr=boolean
  eMduMotCtrl : Inport  Port=3
  s16Vu : Inport  Port=4  OutDataTypeStr=int16
  s16Vv : Inport  Port=5  OutDataTypeStr=int16
  s16Vw : Inport  Port=6  OutDataTypeStr=int16
  Constant2 : Constant  Value=0  OutDataTypeStr=int16
  Constant3 : Constant  OutDataTypeStr=int16
  Constant4 : Constant  Value=2  OutDataTypeStr=int16
  Enumerated Constant : simulink/Sources/Enumerated Constant  OutDataTypeStr=Enum: e_motorstate_t  Value=e_motorstate_t.MOTOR_STATE_OFF  SampleTime=inf
  Enumerated Constant1 : simulink/Sources/Enumerated Constant  OutDataTypeStr=Enum: e_motorstate_t  Value=e_motorstate_t.MOTOR_STATE_FINAL_OFF  SampleTime=inf
  FINAL_OFF : Subsystem  TreatAsAtomicUnit=on
  If : If  NumInputs=2  IfExpression=u1 == 0  ElseIfExpressions=u1 == 10,u2 >= 0
  Merge{,1..3} (4 alike) : Merge  Inputs=4
  Relational Operator1 : RelationalOperator  Operator===  OutDataTypeStr=boolean  RndMeth=Simplest  InputSameDT=off
  Relational Operator2 : RelationalOperator  Operator===  OutDataTypeStr=boolean  RndMeth=Simplest  InputSameDT=off
  STATE_OFF : Subsystem  TreatAsAtomicUnit=on
  SectorDetectionPart1 : Subsystem  TreatAsAtomicUnit=on
  SectorDetectionPart2 : Subsystem  TreatAsAtomicUnit=on
  Switch1 : Switch  Criteria=u2 ~= 0  SaturateOnIntegerOverflow=off  InputSameDT=off
  Switch2 : Switch  Criteria=u2 ~= 0  SaturateOnIntegerOverflow=off  InputSameDT=off
  stSvmDutyU : Outport
  u8SvmSector : Outport  Port=2  OutDataTypeStr=uint8
  stSvmDutyV : Outport  Port=3
  stSvmDutyW : Outport  Port=4
  wires:
  If/2 -> FINAL_OFF/Action
  [s16Vw] -> SectorDetectionPart2/3(s16Vw)
  [stSvmDutyVOff] -> Merge2/1
  [s16Vu] -> SectorDetectionPart2/1(s16Vu)
  [u8SvmSectorPart1] -> Merge1/3
  [stSvmDutyUFinalOff] -> Merge/2
  [u8SvmSectorOff] -> Merge1/1
  [s16Vv] -> SectorDetectionPart2/2(s16Vv)
  [stSvmDutyUOff] -> Merge/1
  [u8SvmSectorPart2] -> Merge1/4
  s16Vu/1 -> SectorDetectionPart1/1(s16Vu), [s16Vu]
  [u8SvmSectorFinalOff] -> Merge1/2
  [stSvmDutyVPart1] -> Merge2/3
  [stSvmDutyVFinalOff] -> Merge2/2
  SectorDetectionPart2/3(stSvmDutyV) -> [stSvmDutyVPart2]
  [stSvmDutyVPart2] -> Merge2/4
  [stSvmDutyUPart1] -> Merge/3
  [stSvmDutyUPart2] -> Merge/4
  eStMotor/1 -> Relational Operator1/1, Relational Operator2/1
  Enumerated Constant/1 -> Relational Operator1/2
  If/3 -> SectorDetectionPart1/Action
  Enumerated Constant1/1 -> Relational Operator2/2
  [stSvmDutyWOff] -> Merge3/1
  [stSvmDutyWFinalOff] -> Merge3/2
  SectorDetectionPart2/1(stSvmDutyU) -> [stSvmDutyUPart2]
  [stSvmDutyWPart1] -> Merge3/3
  [stSvmDutyWPart2] -> Merge3/4
  Switch1/1 -> If/1
  Merge1/1 -> u8SvmSector/1
  Merge2/1 -> stSvmDutyV/1
  SectorDetectionPart1/3(stSvmDutyV) -> [stSvmDutyVPart1]
  STATE_OFF/2(u8SvmSector) -> [u8SvmSectorOff]
  Merge/1 -> stSvmDutyU/1
  If/1 -> STATE_OFF/Action
  Relational Operator1/1 -> Switch1/2
  SectorDetectionPart1/4(stSvmDutyW) -> [stSvmDutyWPart1]
  STATE_OFF/3(stSvmDutyV) -> [stSvmDutyVOff]
  Constant3/1 -> Switch2/1
  If/4 -> SectorDetectionPart2/Action
  Relational Operator2/1 -> Switch2/2
  SectorDetectionPart1/2(u8SvmSector) -> [u8SvmSectorPart1]
  STATE_OFF/1(stSvmDutyU) -> [stSvmDutyUOff]
  Constant4/1 -> Switch2/3
  Merge3/1 -> stSvmDutyW/1
  Constant2/1 -> Switch1/1
  s16Vv/1 -> [s16Vv], SectorDetectionPart1/2(s16Vv)
  Switch2/1 -> Switch1/3
  s16Vw/1 -> [s16Vw], If/2
  bActModeHw/1 -> FINAL_OFF/1(b_hwt_mode_active)
  eMduMotCtrl/1 -> [eMduMotCtrl], SectorDetectionPart1/4(eMduMotCtrl)
  [s16Vw] -> SectorDetectionPart1/3(s16Vw)
  FINAL_OFF/1(stSvmDutyU) -> [stSvmDutyUFinalOff]
  FINAL_OFF/2(u8SvmSector) -> [u8SvmSectorFinalOff]
  FINAL_OFF/3(stSvmDutyV) -> [stSvmDutyVFinalOff]
  FINAL_OFF/4(stSvmDutyW) -> [stSvmDutyWFinalOff]
  STATE_OFF/4(stSvmDutyW) -> [stSvmDutyWOff]
  SectorDetectionPart2/2(u8SvmSector) -> [u8SvmSectorPart2]
  SectorDetectionPart2/4(stSvmDutyW) -> [stSvmDutyWPart2]
  SectorDetectionPart1/1(stSvmDutyU) -> [stSvmDutyUPart1]
  [eMduMotCtrl] -> SectorDetectionPart2/4(eMduMotCtrl)

== system Foc/FieldOrientedControl/SetDutyCycle/SetDuty ==
  stSvmDutyU : Inport
  u8SvmSector : Inport  Port=2  OutDataTypeStr=uint8
  stSvmDutyV : Inport  Port=3
  stSvmDutyW : Inport  Port=4
  Add1 : Sum
  Add12 : Sum  Inputs=+-
  Add13 : Sum  Inputs=+-
  Add2 : Sum
  Bus Creator : BusCreator  Inputs=DesiredPwm_U,DesiredPwm_V,DesiredPwm_W
  Bus Creator1 : BusCreator  Inputs=2
  Bus Creator3 : BusCreator  Inputs=2
  Bus Selector : BusSelector  OutputSignals=u16AdcTrigTick1,u16AdcTrigTick2
  Bus Selector1 : BusSelector  OutputSignals=PwmShiftRiseLong,PwmShiftRiseMed,u16TickShiftV,u16TickShiftU,u16TickShiftW
  Constant : Constant  Value=CCU6_T12PERIOD/2
  Constant15 : Constant  Value=CCU_PWM_PERIOD_TICKS_HALF
  Constant20 : Constant  Value=MIN_SAMPLE_TIME_DEFAULT
  Constant21 : Constant  Value=CCU_PWM_PERIOD_TICKS_HALF
  Constant22 : Constant  Value=MIN_SAMPLE_TIME_DEFAULT
  Constant3 : Constant  Value=cal_bActHwMode
  Constant4 : Constant  Value=false
  Constant5 : Constant  Value=cal_u16AdcTriggerOffset  OutDataTypeStr=uint16
  Default : Subsystem  TreatAsAtomicUnit=on
  Merge : Merge  Inputs=7
  Product : Product  OutDataTypeStr=uint16
  Product1 : Product  OutDataTypeStr=uint16
  Product2 : Product  OutDataTypeStr=uint16
  Relational Operator : RelationalOperator  Operator===  OutDataTypeStr=boolean  RndMeth=Simplest  InputSameDT=off
  Sector1 : Subsystem  TreatAsAtomicUnit=on
  Sector2 : Subsystem  TreatAsAtomicUnit=on
  Sector3 : Subsystem  TreatAsAtomicUnit=on
  Sector4 : Subsystem  TreatAsAtomicUnit=on
  Sector5 : Subsystem  TreatAsAtomicUnit=on
  Sector6 : Subsystem  TreatAsAtomicUnit=on
  Switch : Switch  Criteria=u2 ~= 0  SaturateOnIntegerOverflow=off  InputSameDT=off
  Switch Case : SwitchCase  CaseConditions={1,2,3,4,5,6}
  u16AdcTrigTick1 : Outport  OutDataTypeStr=uint16
  u16AdcTrigTick2 : Outport  Port=2  OutDataTypeStr=uint16
  u16TickShiftV : Outport  Port=3  OutDataTypeStr=uint16
  u16TickShiftU : Outport  Port=4  OutDataTypeStr=uint16
  u16TickShiftW : Outport  Port=5  OutDataTypeStr=uint16
  wires:
  Constant4/1 -> Relational Operator/2
  [DesiredPwm] -> Sector6/1(DesiredPwm)
  stSvmDutyU/1 -> Product/2
  Sector3/1(Bus3) -> Merge/3
  Constant5/1 -> Add2/1, Add1/2
  Sector2/1(Bus2) -> Merge/2
  u8SvmSector/1 -> Switch Case/1
  Switch Case/1 -> Sector1/Action
  [DesiredPwm] -> Sector1/1(DesiredPwm)
  Constant/1 -> Product1/1, Product2/1, Product/1
  stSvmDutyV/1 -> Product1/2
  [DesiredPwm] -> Default/1(DesiredPwm)
  Default/1(BusDefault) -> Merge/7
  Product/1 -> Bus Creator/1  "DesiredPwm_U"
  Product1/1 -> Bus Creator/2  "DesiredPwm_V"
  Product2/1 -> Bus Creator/3  "DesiredPwm_W"
  [DesiredPwm] -> Sector2/1(DesiredPwm)
  Add12/1 -> Bus Creator3/1  "u16AdcTrigTick1"
  [DesiredPwm] -> Sector3/1(DesiredPwm)
  Switch Case/3 -> Sector3/Action
  Switch Case/2 -> Sector2/Action
  Switch Case/5 -> Sector5/Action
  Switch Case/4 -> Sector4/Action
  Switch Case/7 -> Default/Action
  Switch Case/6 -> Sector6/Action
  Constant22/1 -> Add13/2
  [DesiredPwm] -> Sector4/1(DesiredPwm)
  Add13/1 -> Bus Creator3/2  "u16AdcTrigTick2"
  [DesiredPwm] -> Sector5/1(DesiredPwm)
  Sector5/1(Bus5) -> Merge/5
  Bus Creator/1 -> [DesiredPwm]
  Sector1/1(Bus1) -> Merge/1
  Bus Selector/1 -> u16AdcTrigTick1/1  "<u16AdcTrigTick1>"
  Sector4/1(Bus4) -> Merge/4
  Add1/1 -> Bus Creator1/1  "u16AdcTrigTick1"
  Sector6/1(Bus6) -> Merge/6
  Merge/1 -> Bus Selector1/1
  Bus Selector1/1 -> Add1/1  "<PwmShiftRiseLong>"
  Bus Selector1/2 -> Add2/2  "<PwmShiftRiseMed>"
  Bus Selector1/3 -> u16TickShiftV/1  "<u16TickShiftV>"
  Bus Selector1/4 -> u16TickShiftU/1  "<u16TickShiftU>"
  Bus Selector1/5 -> u16TickShiftW/1  "<u16TickShiftW>"
  Constant15/1 -> Add12/1
  Constant20/1 -> Add12/2
  Constant21/1 -> Add13/1
  Add2/1 -> Bus Creator1/2  "u16AdcTrigTick2"
  Constant3/1 -> Relational Operator/1
  Bus Creator1/1 -> Switch/1
  Relational Operator/1 -> Switch/2
  Bus Creator3/1 -> Switch/3
  Switch/1 -> Bus Selector/1
  Bus Selector/2 -> u16AdcTrigTick2/1  "<u16AdcTrigTick2>"
  stSvmDutyW/1 -> Product2/2

== system Foc/FieldOrientedControl/CurrentControl/MOTOR_STATE_ALIGNMENT/EnableDriver ==
  s16AngleParkLast : Inport  OutDataTypeStr=int16
  Bus Creator : BusCreator  Inputs=4
  Constant : Constant  Value=true  OutDataTypeStr=boolean
  Constant1 : Constant  Value=0  OutDataTypeStr=int16
  Constant2 : Constant  Value=0  OutDataTypeStr=int16
  foc_state : Outport
  wires:
  s16AngleParkLast/1 -> Bus Creator/1  "s16AnglePark"
  Constant1/1 -> Bus Creator/2  "s16Vd"
  Constant2/1 -> Bus Creator/3  "s16Vq"
  Constant/1 -> Bus Creator/4  "bEnMotorDriver"
  Bus Creator/1 -> foc_state/1

== system Foc/FieldOrientedControl/CurrentControl/MOTOR_STATE_ALIGNMENT/SetPiController ==
  s16Id : Inport  OutDataTypeStr=int16
  s16Iq : Inport  Port=2  OutDataTypeStr=int16
  bEnMotorDriverLast : Inport  Port=3  OutDataTypeStr=boolean
  s16IdRef : Inport  Port=4  OutDataTypeStr=int16
  s16IqRef : Inport  Port=5  OutDataTypeStr=int16
  IqPiBus : Inport  Port=6
  IdPiBus : Inport  Port=7
  Bus Creator : BusCreator  Inputs=4
  Constant : Constant  Value=0  VectorParams1D=off  OutDataTypeStr=int16
  PiCtrl_Calc_D : Subsystem
  PiCtrl_Calc_q : Subsystem
  foc_state : Outport
  wires:
  s16Id/1 -> PiCtrl_Calc_D/1(s16Id)
  PiCtrl_Calc_q/1(s16Vq) -> Bus Creator/3  "s16Vq"
  s16Iq/1 -> PiCtrl_Calc_q/1(s16Iq)
  Constant/1 -> Bus Creator/1  "s16AnglePark"
  PiCtrl_Calc_D/1(s16Vd) -> Bus Creator/2  "s16Vd"
  bEnMotorDriverLast/1 -> Bus Creator/4  "bEnMotorDriver"
  Bus Creator/1 -> foc_state/1
  s16IdRef/1 -> PiCtrl_Calc_D/2(s16IdRef)
  s16IqRef/1 -> PiCtrl_Calc_q/2(s16IqRef)
  IqPiBus/1 -> PiCtrl_Calc_q/3(IqPiBus)
  IdPiBus/1 -> PiCtrl_Calc_D/3(IdPiBus)

== system Foc/FieldOrientedControl/CurrentControl/MOTOR_STATE_BACK/PiCtrl_Calc_D ==
  s16Id : Inport  OutDataTypeStr=int16
  s16IdRef : Inport  Port=2  OutDataTypeStr=int16
  IdPiBus : Inport  Port=3
  Bus Selector : BusSelector  OutputSignals=s16IdKi,s16IdMaxOut,s8IdFacKi,s16IdMinOut,s16IdKp,s8IdFacKp
  PiControl : Subsystem  TreatAsAtomicUnit=on
  s16Vd : Outport  OutDataTypeStr=int16
  wires:
  s16Id/1 -> PiControl/2(s16InMeas)
  PiControl/1(s16Out) -> s16Vd/1
  s16IdRef/1 -> PiControl/1(s16InRef)
  IdPiBus/1 -> Bus Selector/1
  Bus Selector/1 -> PiControl/3(s16Ki)  "<s16IdKi>"
  Bus Selector/2 -> PiControl/4(s16OutMax)  "<s16IdMaxOut>"
  Bus Selector/3 -> PiControl/5(s8FacKi)  "<s8IdFacKi>"
  Bus Selector/4 -> PiControl/6(s16OutMin)  "<s16IdMinOut>"
  Bus Selector/5 -> PiControl/7(s16Kp)  "<s16IdKp>"
  Bus Selector/6 -> PiControl/8(s8FacKp)  "<s8IdFacKp>"

== system Foc/FieldOrientedControl/CurrentControl/MOTOR_STATE_BACK/PiCtrl_Calc_Q  ==
  s16Iq : Inport  OutDataTypeStr=int16
  s16IqRef : Inport  Port=2  OutDataTypeStr=int16
  IqPiBus : Inport  Port=3
  Bus Selector : BusSelector  OutputSignals=s16IqKi,s16IqMaxOut,s8IqFacKi,s16IqMinOut,s16IqKp,s8IqFacKp
  PiControl : Subsystem  TreatAsAtomicUnit=on
  s16Vq : Outport  OutDataTypeStr=int16
  wires:
  s16Iq/1 -> PiControl/2(s16InMeas)
  PiControl/1(s16Out) -> s16Vq/1
  s16IqRef/1 -> PiControl/1(s16InRef)
  IqPiBus/1 -> Bus Selector/1
  Bus Selector/1 -> PiControl/3(s16Ki)  "<s16IqKi>"
  Bus Selector/2 -> PiControl/4(s16OutMax)  "<s16IqMaxOut>"
  Bus Selector/3 -> PiControl/5(s8FacKi)  "<s8IqFacKi>"
  Bus Selector/4 -> PiControl/6(s16OutMin)  "<s16IqMinOut>"
  Bus Selector/5 -> PiControl/7(s16Kp)  "<s16IqKp>"
  Bus Selector/6 -> PiControl/8(s8FacKp)  "<s8IqFacKp>"

== system Foc/FieldOrientedControl/CurrentControl/MOTOR_STATE_BACK/parkangle_cal ==
  eDirRun : Inport
  u32SpdRamp : Inport  Port=2  OutDataTypeStr=uint32
  s16AngleParkLast : Inport  Port=3  OutDataTypeStr=int16
  Compare To Constant : simulink/Logic and Bit Operations/Compare To Constant  relop===  const=e_running_dir_t.CLOCKWISE  OutDataTypeStr=boolean
  ParkAngleCcw : Subsystem
  ParkAngleCw : Subsystem
  Switch : Switch  Criteria=u2 > Threshold  SaturateOnIntegerOverflow=off  InputSameDT=off
  s16AnglePark : Outport  OutDataTypeStr=int16
  wires:
  u32SpdRamp/1 -> [u32SpdRamp]
  s16AngleParkLast/1 -> [s16AngleParkLast]
  [u32SpdRamp] -> ParkAngleCw/1(u32SpdRamp)
  [s16AngleParkLast] -> ParkAngleCw/2(s16AngleParkLast)
  ParkAngleCw/1(s16AnglePark) -> Switch/1
  [s16AngleParkLast] -> ParkAngleCcw/2(s16AngleParkLast)
  Switch/1 -> s16AnglePark/1
  eDirRun/1 -> Compare To Constant/1
  [u32SpdRamp] -> ParkAngleCcw/1(u32SpdRamp)
  Compare To Constant/1 -> Switch/2
  ParkAngleCcw/1(s16AnglePark) -> Switch/3

== system Foc/FieldOrientedControl/CurrentControl/MOTOR_STATE_BRAKE/EnableDriver ==
  s16AngleParkLast : Inport  OutDataTypeStr=int16
  Bus Creator : BusCreator  Inputs=4
  Constant : Constant  Value=true  OutDataTypeStr=boolean
  Constant1 : Constant  Value=0  OutDataTypeStr=int16
  Constant2 : Constant  Value=0  OutDataTypeStr=int16
  foc_state : Outport
  wires:
  s16AngleParkLast/1 -> Bus Creator/1  "s16AnglePark"
  Constant1/1 -> Bus Creator/2  "s16Vd"
  Constant2/1 -> Bus Creator/3  "s16Vq"
  Constant/1 -> Bus Creator/4  "bEnMotorDriver"
  Bus Creator/1 -> foc_state/1

== system Foc/FieldOrientedControl/CurrentControl/MOTOR_STATE_BRAKE/SetPiController ==
  s16Id : Inport  OutDataTypeStr=int16
  s16Iq : Inport  Port=2  OutDataTypeStr=int16
  bEnMotorDriverLast : Inport  Port=3  OutDataTypeStr=boolean
  s16IdRef : Inport  Port=4  OutDataTypeStr=int16
  s16IqRef : Inport  Port=5  OutDataTypeStr=int16
  IqPiBus : Inport  Port=6
  IdPiBus : Inport  Port=7
  Bus Creator : BusCreator  Inputs=4
  Constant : Constant  Value=0  VectorParams1D=off  OutDataTypeStr=int16
  PiCtrl_Calc_D : Subsystem
  PiCtrl_Calc_q : Subsystem
  foc_state : Outport
  wires:
  s16Id/1 -> PiCtrl_Calc_D/1(s16Id)
  PiCtrl_Calc_q/1(s16Vq) -> Bus Creator/3  "s16Vq"
  s16Iq/1 -> PiCtrl_Calc_q/1(s16Iq)
  Constant/1 -> Bus Creator/1  "s16AnglePark"
  PiCtrl_Calc_D/1(s16Vd) -> Bus Creator/2  "s16Vd"
  bEnMotorDriverLast/1 -> Bus Creator/4  "bEnMotorDriver"
  Bus Creator/1 -> foc_state/1
  s16IdRef/1 -> PiCtrl_Calc_D/2(s16IdRef)
  IdPiBus/1 -> PiCtrl_Calc_D/3(IdPiBus)
  s16IqRef/1 -> PiCtrl_Calc_q/2(s16IqRef)
  IqPiBus/1 -> PiCtrl_Calc_q/3(IqPiBus)

== system Foc/FieldOrientedControl/CurrentControl/MOTOR_STATE_CLOSED_LOOP/ PiCtrl_Calc ==
  s16Id : Inport  OutDataTypeStr=int16
  s16IdRef : Inport  Port=2  OutDataTypeStr=int16
  IdPiBus : Inport  Port=3
  " CalcVqMax" : Subsystem  Commented=on
  Bus Selector : BusSelector  OutputSignals=s16IdKi,s16IdMaxOut,s8IdFacKi,s16IdMinOut,s16IdKp,s8IdFacKp
  PiControl : Subsystem  TreatAsAtomicUnit=on
  s16Vd : Outport  OutDataTypeStr=int16
  wires:
  s16Id/1 -> PiControl/2(s16InMeas)
  PiControl/1(s16Out) -> s16Vd/1
  s16IdRef/1 -> PiControl/1(s16InRef)
  Bus Selector/1 -> PiControl/3(s16Ki)  "<s16IdKi>"
  Bus Selector/2 -> PiControl/4(s16OutMax)  "<s16IdMaxOut>"
  Bus Selector/3 -> PiControl/5(s8FacKi)  "<s8IdFacKi>"
  Bus Selector/4 -> PiControl/6(s16OutMin)  "<s16IdMinOut>"
  Bus Selector/5 -> PiControl/7(s16Kp)  "<s16IdKp>"
  Bus Selector/6 -> PiControl/8(s8FacKp)  "<s8IdFacKp>"
  IdPiBus/1 -> Bus Selector/1
